simulink model "BoostConverterVoltageGain_w_r_t_DutyCycle"  (R2021a)
settings: Solver=VariableStepAuto  StartTime=0.0  StopTime=0.1  RelTol=1e-3
libraries: spsCurrentMeasurementLib x4, spsVoltageMeasurementLib x4, spsSeriesRLCBranchLib x3, spsDCVoltageSourceLib x1, spsDiodeLib x1, spsMosfetLib x1, spspowerguiLib x1
settings Model: Creator=EREN-PC  LastModifiedBy=EREN-PC

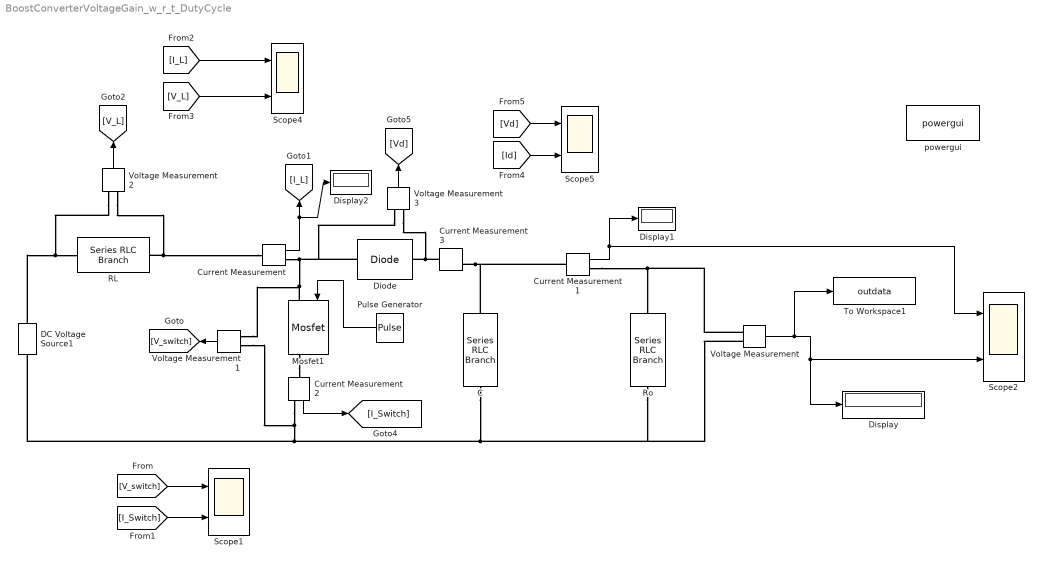
== system BoostConverterVoltageGain_w_r_t_DutyCycle ==
  C : spsSeriesRLCBranchLib/Series RLC Branch  LConnTagsString=__new0  RConnTagsString=__new0  BranchType=C  Resistance=1  Inductance=1e-3  SetiL0=off  InitialCurrent=0  Capacitance=1e-5  Setx0=off  InitialVoltage=0  Measurements=None
  Current Measurement{,1..3} (4 alike) : spsCurrentMeasurementLib/Current Measurement  PhasorSimulation=off  OutputType=Complex  PSBequivalent=0
  DC Voltage Source1 : spsDCVoltageSourceLib/DC Voltage Source  Amplitude=5  Measurements=None
  Diode : spsDiodeLib/Diode  Ron=0.001  Lon=0  Vf=0  IC=0  UseSnubber=0  Rs=500  Cs=250e-9  Measurements=off
  Display : Display
  Display1 : Display
  Display2 : Display
  Mosfet1 : spsMosfetLib/Mosfet  Ron=0.1  Lon=0  Rd=0.01  Vfd=0  IC=0  Rs=1e5  Cs=inf  Measurements=on
  Pulse Generator : DiscretePulseGenerator  PulseType=Time based  Period=1/300000  PulseWidth=10
  RL : spsSeriesRLCBranchLib/Series RLC Branch  LConnTagsString=__new0  RConnTagsString=__new0  BranchType=L  Resistance=1  Inductance=5e-5  SetiL0=off  InitialCurrent=0  Capacitance=1e-6  Setx0=off  InitialVoltage=0  Measurements=None
  Ro : spsSeriesRLCBranchLib/Series RLC Branch  LConnTagsString=__new0  RConnTagsString=__new0  BranchType=R  Resistance=256  Inductance=1e-3  SetiL0=off  InitialCurrent=0  Capacitance=1e-6  Setx0=off  InitialVoltage=0  Measurements=None
  Scope{1..2,4..5} (4 alike) : Scope  NumInputPorts=2
  To Workspace1 : ToWorkspace  VariableName=outdata  SampleTime=-1
  Voltage Measurement{,1..3} (4 alike) : spsVoltageMeasurementLib/Voltage Measurement  PhasorSimulation=off  OutputType=Complex  PSBequivalent=0
  powergui : spspowerguiLib/powergui  Priority=1  SimulationMode=Continuous  SampleTime=5e-7  frequency=60  Iterations=50  frequencyindice=0  Pbase=100e6  ErrMax=1e-4  UnitsV=kV  UnitsW=MW  buscounter=0  FunctionMessages=off  echomessages=off  EnableUseOfTLC=off  CurrentSourceSwitches=off  DisableSnubberDevices=off  DisableRonSwitches=off  DisableVfSwitches=off  DisplayEquations=off  AutomaticDiscreteSolvers=off  SolverType=Tustin/Backward Euler (TBE)  Interpol=off  ExternalGateDelay=off  methode=off  Ts=100  x0status=blocks  SPID=on  SwTol=0  HookPort=off  NonlinearTolerance=1e-4  nMaxIteration=100  ContinueOnMaxIteration=off  RestoreLinks=warning  ResistiveCurrentMeasurement=off  Frange=[0:2:500]  Ylog=off  Xlog=on  ShowGrid=off  save=off  variable=ZData  structure=0  ZoomFFT=off  StartTime=0.0  cycles=1  DisplayStyle=1  fundamental=60  FreqAxis=off  MaxFrequency=1000  frequencyindicesteady=1  RmsSteady=1  display=off
  wires:
  [I_L] -> Scope4/1
  Voltage Measurement1/1 -> [V_switch]
  Current Measurement2/1 -> [I_Switch]
  Voltage Measurement/1 -> To Workspace1/1, Scope2/2, Display/1
  [V_switch] -> Scope1/1
  [V_L] -> Scope4/2
  Voltage Measurement2/1 -> [V_L]
  [I_Switch] -> Scope1/2
  Voltage Measurement3/1 -> [Vd]
  Current Measurement1/1 -> Scope2/1, Display1/1
  [Vd] -> Scope5/1
  Current Measurement/1 -> Display2/1, [I_L]
  Pulse Generator/1 -> Mosfet1/1
  [Id] -> Scope5/2
  connections:
  Current Measurement2/RConn1 -- Voltage Measurement/LConn2 -- Ro/RConn1 -- C/RConn1 -- DC Voltage Source1/LConn1 -- Voltage Measurement1/LConn2
  Voltage Measurement1/LConn1 -- Mosfet1/LConn1 -- Current Measurement/RConn1 -- Diode/LConn1 -- Voltage Measurement3/LConn1
  Current Measurement3/RConn1 -- C/LConn1 -- Current Measurement1/LConn1
  Current Measurement1/RConn1 -- Voltage Measurement/LConn1 -- Ro/LConn1
  Voltage Measurement2/LConn1 -- DC Voltage Source1/RConn1 -- RL/LConn1
  Diode/RConn1 -- Current Measurement3/LConn1 -- Voltage Measurement3/LConn2
  Mosfet1/RConn1 -- Current Measurement2/LConn1
  Voltage Measurement2/LConn2 -- Current Measurement/LConn1 -- RL/RConn1
